simulink model "Mip_Balance_Demo_2019B"  (R2019b)
settings: Solver=FixedStepAuto  StartTime=0.0  StopTime=inf  RelTol=1e-3
undefined symbols (not defined in the file): DiscIntNeverNeededParam
libraries: bbblueSensorLib x3, simulink x2, bbblueActuatorLib x2, bbblueBasicLib x2, simulink_extras x1
settings Model: SimulationMode=external  Creator=ktalke  LastModifiedBy=ricardo
settings SolverCC: PositivePriorityOrder=on  AutoInsertRateTranBlk=on
settings DataIOCC: ReturnWorkspaceOutputs=off
settings OptimizationCC: EnhancedBackFolding=on  PassReuseOutputArgsAs=Individual arguments  MaxStackSize=64  OptimizeBlockOrder=speed  DifferentSizesBufferReuse=on  OptimizationCustomize=off  EfficientTunableParamExpr=on
settings DebuggingCC: ParameterTunabilityLossMsg=error  ArithmeticOperatorsInVariantConditions=warning
settings HardwareCC: ProdBitPerPointer=32  ProdBitPerSizeT=32  ProdBitPerPtrDiffT=32  ProdLargestAtomicInteger=Long  ProdLargestAtomicFloat=Double  ProdWordSize=32  ProdHWDeviceType=ARM Compatible->ARM Cortex
settings SFSimCC: SimUseLocalCustomCode=off  MATLABDynamicMemAlloc=off  CustomCodeUndefinedFunction=UseInterfaceOnly
settings RTWCC: SystemTargetFile=ert.tlc  HardwareBoard=BeagleBone Blue  TLCOptions="-aInlineSetEventsForThisBaseRateFcn=TLC_FALSE -aSuppressMultiTaskScheduler=TLC_FALSE  -aRateBasedStepFcn=0"  TemplateMakefile=ert_default_tmf  RTWUseLocalCustomCode=off  Toolchain=GNU GCC BeagleBone Blue  IncludeHyperlinkInReport=on
settings CodeAppCC: ForceParamTrailComments=on  IgnoreCustomStorageClasses=off  OperatorAnnotations=on  SimulinkDataObjDesc=on  SFDataObjDesc=on  InsertBlockDesc=on
settings ERTTargetCC: SupportVariableSizeSignals=on

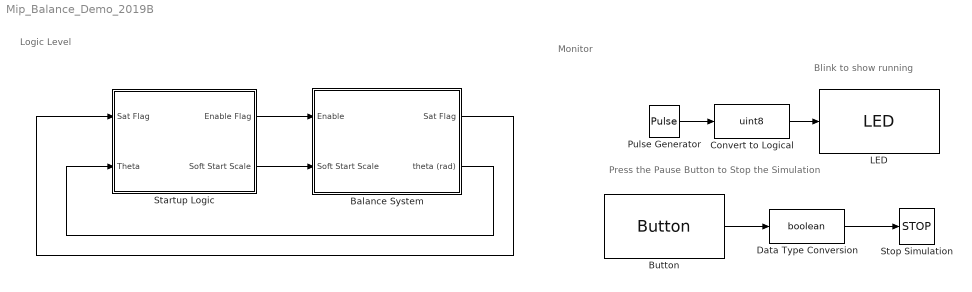
== system Mip_Balance_Demo_2019B ==
  note: Press the Pause Button to Stop the Simulation
  note: Logic Level
  note: Monitor
  note: Blink to show running
  Balance System : Subsystem  TreatAsAtomicUnit=on
  Button : bbblueBasicLib/Button  Button=Pause  SampleTime=0.1  SimulateUsing=Code generation
      settings: SourceProductName=Simulink Coder Support Package for BeagleBone Blue Hardware
  Convert to Logical : DataTypeConversion  OutDataTypeStr=uint8
  Data Type Conversion : DataTypeConversion  OutDataTypeStr=boolean
  LED : bbblueBasicLib/LED  LED=Green
      settings: SourceProductName=Simulink Coder Support Package for BeagleBone Blue Hardware
  Pulse Generator : DiscretePulseGenerator  Period=10  PulseWidth=5  SampleTime=0.1
  Startup Logic : Subsystem
  Stop Simulation : Stop
  wires:
  Button/1 -> Data Type Conversion/1
  Startup Logic/2(Soft Start Scale) -> Balance System/2(Soft Start Scale)
  Pulse Generator/1 -> Convert to Logical/1
  Balance System/1(Sat Flag) -> Startup Logic/1(Sat Flag)
  Balance System/2(theta (rad)) -> Startup Logic/2(Theta)
  Data Type Conversion/1 -> Stop Simulation/1
  Startup Logic/1(Enable Flag) -> Balance System/1(Enable)
  Convert to Logical/1 -> LED/1

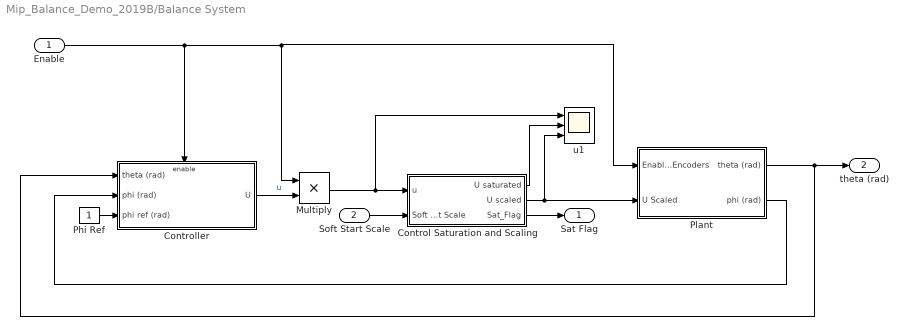
== system Mip_Balance_Demo_2019B/Balance System ==
  Enable : Inport
  Soft Start Scale : Inport  Port=2
  Control Saturation and Scaling : Subsystem
  Controller : Subsystem
  Multiply : Product
  Phi Ref : Constant
  Plant : Subsystem
  u1 : Scope  NumInputPorts=3
  Sat Flag : Outport  VectorParamsAs1DForOutWhenUnconnected=off
  theta (rad) : Outport  Port=2  VectorParamsAs1DForOutWhenUnconnected=off
  wires:
  Phi Ref/1 -> Controller/3(phi ref (rad))
  Control Saturation and Scaling/1(U saturated) -> u1/2
  Control Saturation and Scaling/2(U scaled) -> Plant/2(U Scaled), u1/3
  Control Saturation and Scaling/3(Sat_Flag) -> Sat Flag/1
  Soft Start Scale/1 -> Control Saturation and Scaling/2(Soft Start Scale)
  Enable/1 -> Controller/Enable, Plant/1(Enable Encoders), Multiply/1
  Plant/1(theta (rad)) -> Controller/1(theta (rad)), theta (rad)/1
  Plant/2(phi (rad)) -> Controller/2(phi (rad))
  Controller/1(U) -> Multiply/2  "u"
  Multiply/1 -> u1/1, Control Saturation and Scaling/1(u)

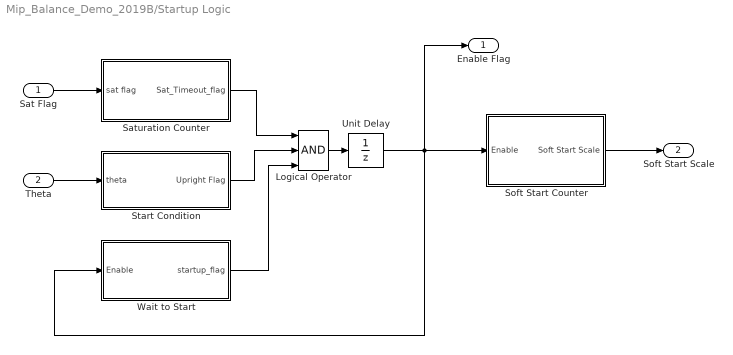
== system Mip_Balance_Demo_2019B/Startup Logic ==
  Sat Flag : Inport
  Theta : Inport  Port=2
  Logical Operator : Logic  Inputs=3  AllPortsSameDT=off  OutDataTypeStr=boolean
  Saturation Counter : Subsystem
  "Soft Start Counter " : Subsystem
  Start Condition : Subsystem
  Unit Delay : UnitDelay  SampleTime=-1  HasFrameUpgradeWarning=on
  Wait to Start : Subsystem
  Enable Flag : Outport  VectorParamsAs1DForOutWhenUnconnected=off
  Soft Start Scale : Outport  Port=2  VectorParamsAs1DForOutWhenUnconnected=off
  wires:
  Wait to Start/1(startup_flag) -> Logical Operator/3
  Logical Operator/1 -> Unit Delay/1
  Start Condition/1(Upright Flag) -> Logical Operator/2
  Saturation Counter/1(Sat_Timeout_flag) -> Logical Operator/1
  "Soft Start Counter "/1(Soft Start Scale) -> Soft Start Scale/1
  Sat Flag/1 -> Saturation Counter/1(sat flag)
  Theta/1 -> Start Condition/1(theta)
  Unit Delay/1 -> Enable Flag/1, "Soft Start Counter "/1(Enable), Wait to Start/1(Enable)

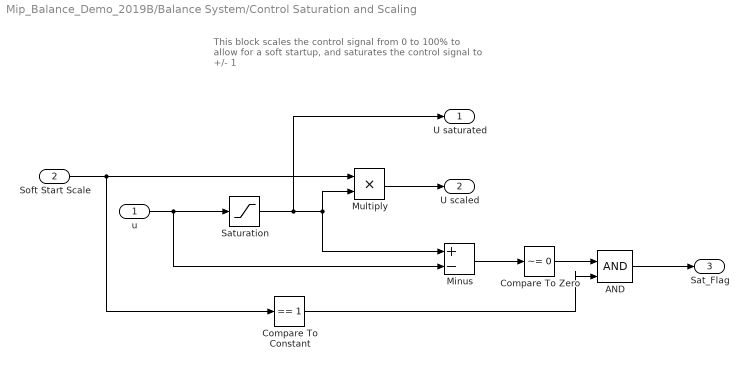
== system Mip_Balance_Demo_2019B/Balance System/Control Saturation and Scaling ==
  note: This block scales the control signal from 0 to 100% to allow for a soft startup, and saturates the control signal to +/- 1
  u : Inport
  Soft Start Scale : Inport  Port=2
  AND : Logic  IconShape=distinctive  AllPortsSameDT=off  OutDataTypeStr=boolean
  Compare To Constant : simulink/Logic and Bit Operations/Compare To Constant  relop===  const=1  OutDataTypeStr=boolean
  Compare To Zero : simulink/Logic and Bit Operations/Compare To Zero  relop=~=  OutDataTypeStr=boolean
  Minus : Sum  Inputs=+-
  Multiply : Product
  Saturation : Saturate  UpperLimit=1  LowerLimit=-1
  U saturated : Outport  VectorParamsAs1DForOutWhenUnconnected=off
  U scaled : Outport  Port=2  OutDataTypeStr=double  PortDimensions=[1 1]  SampleTime=[0.01,0]  VectorParamsAs1DForOutWhenUnconnected=off
  Sat_Flag : Outport  Port=3  VectorParamsAs1DForOutWhenUnconnected=off
  wires:
  u/1 -> Minus/2, Saturation/1
  Minus/1 -> Compare To Zero/1
  Soft Start Scale/1 -> Compare To Constant/1, Multiply/1
  Multiply/1 -> U scaled/1
  Saturation/1 -> U saturated/1, Minus/1, Multiply/2
  Compare To Zero/1 -> AND/1
  Compare To Constant/1 -> AND/2
  AND/1 -> Sat_Flag/1

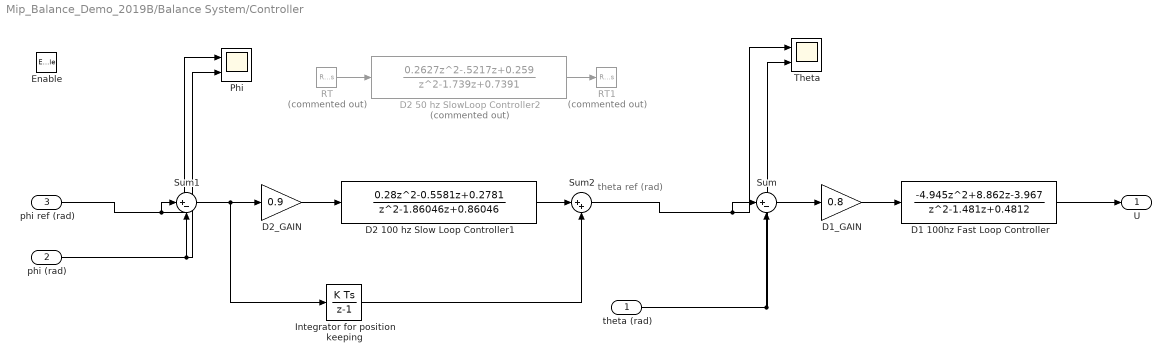
== system Mip_Balance_Demo_2019B/Balance System/Controller ==
  note: theta ref (rad)
  theta (rad) : Inport
  phi (rad) : Inport  Port=2
  phi ref (rad) : Inport  Port=3
  Enable : EnablePort  StatesWhenEnabling=reset
  D1 100hz Fast Loop Controller : DiscreteTransferFcn  Numerator=[-4.945, 8.862, -3.967]  Denominator=[1.000, -1.481, 0.4812]
  D1_GAIN : Gain  Gain=0.8
  D2 100 hz Slow Loop Controller1 : DiscreteTransferFcn  Numerator="[0.28,  -0.5581,  0.2781]"  Denominator="[1.00000,  -1.86046,   0.86046]"
  D2 50 hz SlowLoop Controller2 : DiscreteTransferFcn  Commented=on  Numerator="[0.2627,  -.5217, 0.259]"  Denominator="[1.00000,  -1.739, 0.7391]"  SampleTime=.02
  D2_GAIN : Gain  Gain=0.9
  Integrator for position keeping : DiscreteIntegrator  gainval=.005  SampleTime=-1  ICPrevOutput=DiscIntNeverNeededParam  ICPrevScaledInput=DiscIntNeverNeededParam
  Phi : Scope  NumInputPorts=2
  RT : RateTransition  Commented=on  OutPortSampleTime=0.05
  RT1 : RateTransition  Commented=on  OutPortSampleTime=0.01
  Sum : Sum  Inputs=|+-
  Sum1 : Sum  Inputs=|+-
  Sum2 : Sum  Inputs=|++
  Theta : Scope  NumInputPorts=2
  U : Outport  VectorParamsAs1DForOutWhenUnconnected=off
  wires:
  phi ref (rad)/1 -> Phi/1, Sum1/1
  D1_GAIN/1 -> D1 100hz Fast Loop Controller/1
  theta (rad)/1 -> Theta/2, Sum/2
  phi (rad)/1 -> Phi/2, Sum1/2
  Sum1/1 -> D2_GAIN/1, Integrator for position keeping/1
  Sum/1 -> D1_GAIN/1
  D2_GAIN/1 -> D2 100 hz Slow Loop Controller1/1
  Integrator for position keeping/1 -> Sum2/2
  Sum2/1 -> Theta/1, Sum/1
  D2 50 hz SlowLoop Controller2/1 -> RT1/1
  RT/1 -> D2 50 hz SlowLoop Controller2/1
  D1 100hz Fast Loop Controller/1 -> U/1
  D2 100 hz Slow Loop Controller1/1 -> Sum2/1

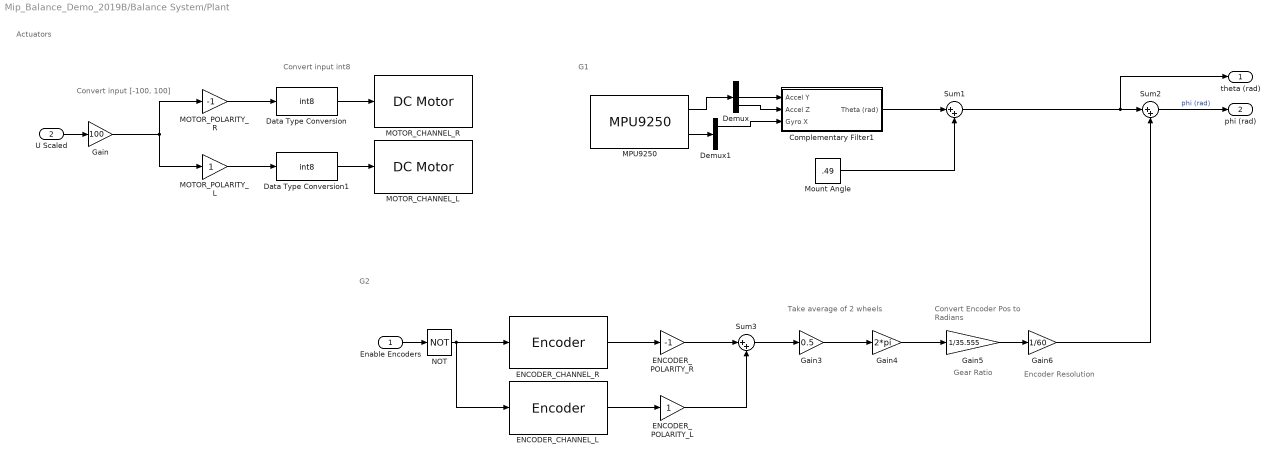
== system Mip_Balance_Demo_2019B/Balance System/Plant ==
  note: G2
  note: G1
  note: Actuators
  note: Convert input
      | [-100, 100]
  note: Convert input
      | int8
  note: Gear Ratio
  note: Encoder
      | Resolution
  note: Convert Encoder Pos
      | to Radians
  note: Take average
      | of 2 wheels
  Enable Encoders : Inport
  U Scaled : Inport  Port=2
  Complementary Filter1 : Subsystem
  Data Type Conversion : DataTypeConversion  OutDataTypeStr=int8  SaturateOnIntegerOverflow=on  RndMeth=Zero
  Data Type Conversion1 : DataTypeConversion  OutDataTypeStr=int8  SaturateOnIntegerOverflow=on  RndMeth=Zero
  Demux : Demux  Outputs=3
  Demux1 : Demux  Outputs=3
  ENCODER_CHANNEL_L : bbblueSensorLib/Encoder  Channel=3  Mode=Reset by external signal  SampleTime=0.01  SimulateUsing=Code generation
      settings: SourceProductName=Simulink Coder Support Package for BeagleBone Blue Hardware
  ENCODER_CHANNEL_R : bbblueSensorLib/Encoder  Channel=2  Mode=Reset by external signal  SampleTime=0.01  SimulateUsing=Code generation
      settings: SourceProductName=Simulink Coder Support Package for BeagleBone Blue Hardware
  ENCODER_POLARITY_L : Gain
  ENCODER_POLARITY_R : Gain  Gain=-1
  Gain : Gain  Gain=100
  Gain3 : Gain  Gain=0.5  OutDataTypeStr=double
  Gain4 : Gain  Gain=2*pi
  Gain5 : Gain  Gain=1/35.555
  Gain6 : Gain  Gain=1/60
  MOTOR_CHANNEL_L : bbblueActuatorLib/DC Motor  index=3  stopaction=Free Spin  SimulateUsing=Code generation
      settings: SourceProductName=Simulink Coder Support Package for BeagleBone Blue Hardware
  MOTOR_CHANNEL_R : bbblueActuatorLib/DC Motor  index=2  stopaction=Free Spin  SimulateUsing=Code generation
      settings: SourceProductName=Simulink Coder Support Package for BeagleBone Blue Hardware
  MOTOR_POLARITY_L : Gain
  MOTOR_POLARITY_R : Gain  Gain=-1
  MPU9250 : bbblueSensorLib/MPU9250  OperationMode=DMP  Accel=on  AngularRate=on  Ak8963Field=off  EulerAngles=off  Quat=off  AccelRange=2G  Acceldlpf=1  GyroRange=250 dps  Gyrodlpf=1  DmpOdr=100 Hz  SampleTime=0.01
      settings: SourceProductName=Simulink Coder Support Package for BeagleBone Blue Hardware  SourceProductBaseCode=SC_BEAGLEBONE_BLUE
  Mount Angle : Constant  Value=.49
  NOT : Logic  Operator=NOT  IconShape=distinctive  AllPortsSameDT=off  OutDataTypeStr=boolean
  Sum1 : Sum  Inputs=|++
  Sum2 : Sum  Inputs=|++
  Sum3 : Sum  Inputs=|++
  theta (rad) : Outport  VectorParamsAs1DForOutWhenUnconnected=off
  phi (rad) : Outport  Port=2  VectorParamsAs1DForOutWhenUnconnected=off
  wires:
  Sum2/1 -> phi (rad)/1  "phi (rad)"
  Gain6/1 -> Sum2/2
  Data Type Conversion1/1 -> MOTOR_CHANNEL_L/1
  MOTOR_POLARITY_R/1 -> Data Type Conversion/1
  Data Type Conversion/1 -> MOTOR_CHANNEL_R/1
  U Scaled/1 -> Gain/1
  MOTOR_POLARITY_L/1 -> Data Type Conversion1/1
  Gain/1 -> MOTOR_POLARITY_R/1, MOTOR_POLARITY_L/1
  Sum1/1 -> theta (rad)/1, Sum2/1
  Mount Angle/1 -> Sum1/2
  Complementary Filter1/1(Theta (rad)) -> Sum1/1
  Enable Encoders/1 -> NOT/1
  Gain5/1 -> Gain6/1
  ENCODER_CHANNEL_R/1 -> ENCODER_POLARITY_R/1
  Sum3/1 -> Gain3/1
  ENCODER_POLARITY_R/1 -> Sum3/1
  NOT/1 -> ENCODER_CHANNEL_L/1, ENCODER_CHANNEL_R/1
  Gain4/1 -> Gain5/1
  ENCODER_CHANNEL_L/1 -> ENCODER_POLARITY_L/1
  ENCODER_POLARITY_L/1 -> Sum3/2
  Gain3/1 -> Gain4/1
  MPU9250/1 -> Demux/1
  MPU9250/2 -> Demux1/1
  Demux/2 -> Complementary Filter1/1(Accel Y)
  Demux/3 -> Complementary Filter1/2(Accel Z)
  Demux1/1 -> Complementary Filter1/3(Gyro X)

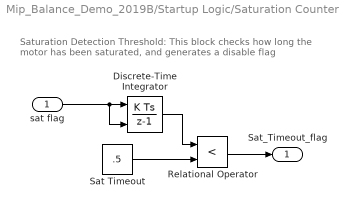
== system Mip_Balance_Demo_2019B/Startup Logic/Saturation Counter ==
  note: Saturation Detection Threshold:
      | This block checks how long the motor has been saturated, and generates a disable flag
  sat flag : Inport
  Discrete-Time Integrator : DiscreteIntegrator  ExternalReset=falling  SampleTime=-1  ICPrevOutput=DiscIntNeverNeededParam  ICPrevScaledInput=DiscIntNeverNeededParam
  Relational Operator : RelationalOperator  Operator=<  OutDataTypeStr=boolean  RndMeth=Simplest
  Sat Timeout : Constant  Value=.5
  Sat_Timeout_flag : Outport  VectorParamsAs1DForOutWhenUnconnected=off
  wires:
  Relational Operator/1 -> Sat_Timeout_flag/1
  Sat Timeout/1 -> Relational Operator/2
  Discrete-Time Integrator/1 -> Relational Operator/1
  sat flag/1 -> Discrete-Time Integrator/1, Discrete-Time Integrator/2

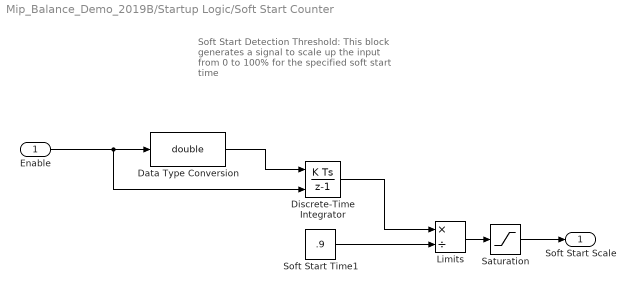
== system Mip_Balance_Demo_2019B/Startup Logic/Soft Start Counter  ==
  note: Soft Start Detection Threshold:
      | This block generates a signal to scale up the input from 0 to 100% for the specified soft start time
  Enable : Inport
  Data Type Conversion : DataTypeConversion  OutDataTypeStr=double
  Discrete-Time Integrator : DiscreteIntegrator  ExternalReset=rising  SampleTime=-1  ICPrevOutput=DiscIntNeverNeededParam  ICPrevScaledInput=DiscIntNeverNeededParam
  Limits : Product  Inputs=*/
  Saturation : Saturate  UpperLimit=1  LowerLimit=0
  Soft Start Time1 : Constant  Value=.9
  Soft Start Scale : Outport  VectorParamsAs1DForOutWhenUnconnected=off
  wires:
  Limits/1 -> Saturation/1
  Discrete-Time Integrator/1 -> Limits/1
  Soft Start Time1/1 -> Limits/2
  Enable/1 -> Data Type Conversion/1, Discrete-Time Integrator/2
  Saturation/1 -> Soft Start Scale/1
  Data Type Conversion/1 -> Discrete-Time Integrator/1

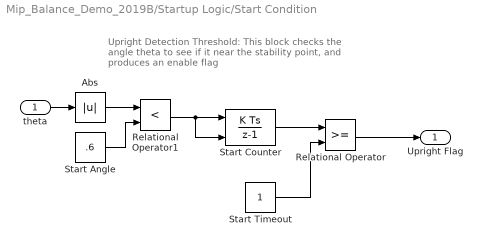
== system Mip_Balance_Demo_2019B/Startup Logic/Start Condition ==
  note: Upright Detection Threshold:
      | This block checks the angle theta to see if it near the stability point, and produces an enable flag
  theta : Inport
  Abs : Abs
  Relational Operator : RelationalOperator  OutDataTypeStr=boolean  RndMeth=Simplest
  Relational Operator1 : RelationalOperator  Operator=<  OutDataTypeStr=boolean  RndMeth=Simplest
  Start Angle : Constant  Value=.6
  Start Counter : DiscreteIntegrator  ExternalReset=falling  SampleTime=-1  RndMeth=Zero  SaturateOnIntegerOverflow=on  UpperSaturationLimit=100  LowerSaturationLimit=-100  ICPrevOutput=DiscIntNeverNeededParam  ICPrevScaledInput=DiscIntNeverNeededParam
  Start Timeout : Constant
  Upright Flag : Outport  VectorParamsAs1DForOutWhenUnconnected=off
  wires:
  theta/1 -> Abs/1
  Start Counter/1 -> Relational Operator/1
  Relational Operator/1 -> Upright Flag/1
  Abs/1 -> Relational Operator1/1
  Start Timeout/1 -> Relational Operator/2
  Relational Operator1/1 -> Start Counter/2, Start Counter/1
  Start Angle/1 -> Relational Operator1/2

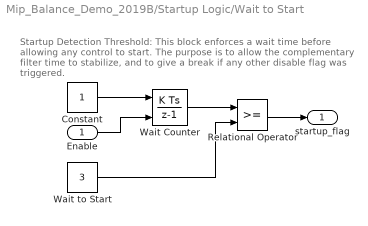
== system Mip_Balance_Demo_2019B/Startup Logic/Wait to Start ==
  note: Startup Detection Threshold:
      | This block enforces a wait time before allowing any control to start. The purpose is to allow the complementary filter time to stabilize, and to give a break if any other disable flag was triggered.
  Enable : Inport
  Constant : Constant
  Relational Operator : RelationalOperator  OutDataTypeStr=boolean  RndMeth=Simplest
  Wait Counter : DiscreteIntegrator  ExternalReset=falling  SampleTime=-1  SaturateOnIntegerOverflow=on  ICPrevOutput=DiscIntNeverNeededParam  ICPrevScaledInput=DiscIntNeverNeededParam
  Wait to Start : Constant  Value=3
  startup_flag : Outport  VectorParamsAs1DForOutWhenUnconnected=off
  wires:
  Wait Counter/1 -> Relational Operator/1
  Constant/1 -> Wait Counter/1
  Wait to Start/1 -> Relational Operator/2
  Relational Operator/1 -> startup_flag/1
  Enable/1 -> Wait Counter/2

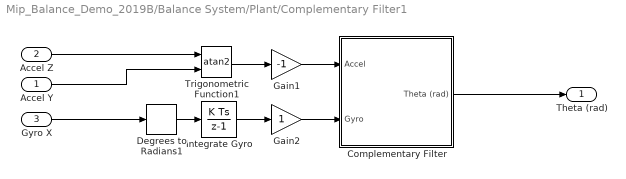
== system Mip_Balance_Demo_2019B/Balance System/Plant/Complementary Filter1 ==
  Accel Y : Inport
  Accel Z : Inport  Port=2
  Gyro X : Inport  Port=3
  Complementary Filter : Subsystem  mask(Complementary Filters){wc=.5, dt=.01}
      mask help:
      | dt - time step
      | wc - time constant
  Degrees to Radians1 : simulink_extras/Transformations/Degrees to Radians
  Gain1 : Gain  Gain=-1
  Gain2 : Gain
  Integrate Gyro : DiscreteIntegrator  SampleTime=-1  ICPrevOutput=DiscIntNeverNeededParam  ICPrevScaledInput=DiscIntNeverNeededParam
  Trigonometric Function1 : Trigonometry  Operator=atan2
  Theta (rad) : Outport  VectorParamsAs1DForOutWhenUnconnected=off
  wires:
  Complementary Filter/1(Theta (rad)) -> Theta (rad)/1
  Accel Z/1 -> Trigonometric Function1/1
  Gyro X/1 -> Degrees to Radians1/1
  Integrate Gyro/1 -> Gain2/1
  Degrees to Radians1/1 -> Integrate Gyro/1
  Accel Y/1 -> Trigonometric Function1/2
  Gain1/1 -> Complementary Filter/1(Accel)
  Trigonometric Function1/1 -> Gain1/1
  Gain2/1 -> Complementary Filter/2(Gyro)

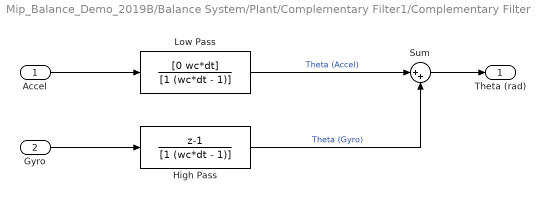
== system Mip_Balance_Demo_2019B/Balance System/Plant/Complementary Filter1/Complementary Filter ==
  Accel : Inport
  Gyro : Inport  Port=2
  "High Pass " : DiscreteTransferFcn  Numerator=[1 -1]  Denominator=[1 (wc*dt - 1)]
  "Low Pass " : DiscreteTransferFcn  Numerator=[0 wc*dt]  Denominator=[1 (wc*dt - 1)]
  Sum : Sum  Inputs=|++
  Theta (rad) : Outport  VectorParamsAs1DForOutWhenUnconnected=off
  wires:
  "High Pass "/1 -> Sum/2  "Theta (Gyro)"
  Accel/1 -> "Low Pass "/1
  Gyro/1 -> "High Pass "/1
  "Low Pass "/1 -> Sum/1  "Theta (Accel)"
  Sum/1 -> Theta (rad)/1
